simulink model "manchestermodelcommblks"  (Simulink 5.1)
settings: Solver=FixedStepDiscrete  SolverMode=SingleTasking  StartTime=0.0  StopTime=50000  RelTol=1e-3
undefined symbols (not defined in the file or in its folder): sigbuilder_block
libraries: fixpt_lib_4 x6, dspsigops x5, commsink2 x2, dspswit3 x1, dspsrcs4 x1, simulink x1, modelsimlib x1
settings Model: Creator=adowd  LastModifiedBy=nsen  ExtModeAutoUpdateStatusClock=off  SaveTime=off  SaveOutput=off  BooleanDataType=on  ProdHWDeviceType=Microprocessor  RTWOptions="-aEnforceIntegerDowncast=1 -aExtMode=0 -aExtModeTesting=0 -aFoldNonRolledExpr=1 -aForceParamTrailComments=0 -aGenerateComments=1 -aGenerateReport=0 -aIgnoreCustomStorageClasses=1 -aIncDataTypeInIds=0 -aIncHierarchyInIds=0 -aInlineInvariantSignals=0 -aInlinedPrmAccess=\"Literals\" -aLocalBlockOutputs=1 -aLogVarNameModifier=\"rt_\" -aMaxRTWIdLen=31 -aPrefixModelToSubsysFcnNames=1 -aRTWVerbose=1 -aRollThreshold=5 -aShowEliminatedStatements=0"

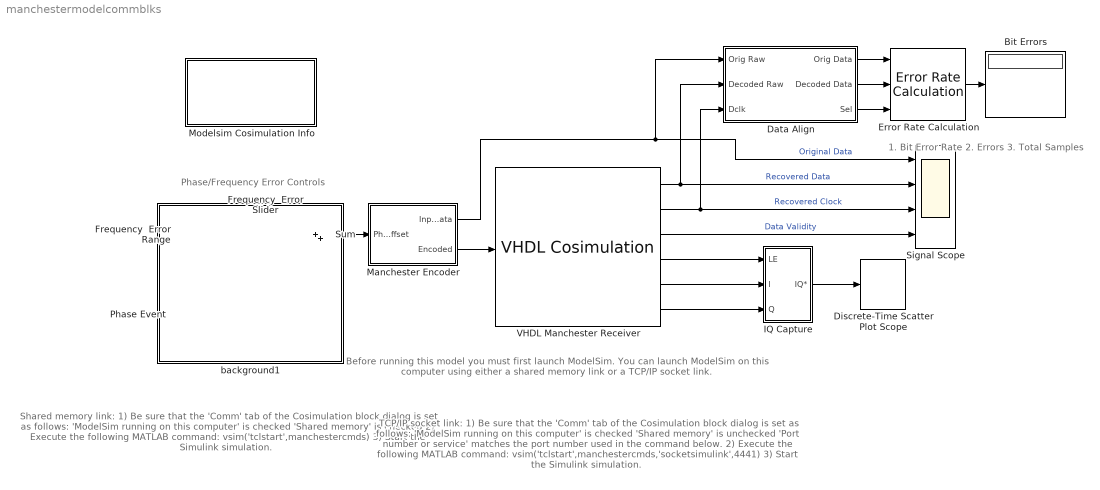
== system manchestermodelcommblks ==
  note: Phase/Frequency Error Controls
  note: 1. Bit Error Rate
      | 2. Errors
      | 3. Total Samples
  note: Before running this model you must first launch ModelSim.
      | You can launch ModelSim on this computer using either a
      | shared memory link or a TCP/IP socket link.
  note: Shared memory link:
      |     1) Be sure that the 'Comm' tab of the Cosimulation block
      |          dialog is set as follows:
      |             'ModelSim running on this computer' is checked
      |             'Shared memory' is checked
      |     2) Execute the following MATLAB command:
      |             vsim('tclstart',manchestercmds)
      |     3) Start the Simulink simulation.
  note: TCP/IP socket link:
      |     1) Be sure that the 'Comm' tab of the Cosimulation block
      |          dialog is set as follows:
      |             'ModelSim running on this computer' is checked
      |             'Shared memory' is unchecked
      |             'Port number or service' matches the port number used
      |                    in the command below.
      |     2) Execute the following MATLAB command:
      |             vsim('tclstart',manchestercmds,'socketsimulink',4441)
      |     3) Start the Simulink simulation.
  Bit Errors : Display
  Data Align : Subsystem
  Discrete-Time Scatter Plot Scope : commsink2/Discrete-Time Scatter Plot Scope  Tag=ScatterPlot  showPlotting=on  sampPerSymb=1  offsetEye=0  numTraces=256  numNewFrames=32  showRendering=on  LineMarkers=d  LineColors=b  fading=on  render=off  AxisGrid=on  showAxes=off  xMin=-0.82  xMax=16.82  yMin=-0.800000000000001  yMax=16.84  inphaseLabel=In-phase Amplitude  quadratureLabel=Quadrature Amplitude  showFigure=off  openScopeAtSimStart=on  FrameNumber=off  FigPos=[360 532 402 402]  figTitle=IQ Measurements  numLinesMax=8  block_type_=scatter
  Error Rate Calculation : commsink2/Error Rate Calculation  N=0  st_delay=0  cp_mode=Select samples from port  subframe=[]  PMode=Port  WsName=ErrorVec  RsMode2=off  stop=off  numErr=100  maxBits=1e6
  Frequency  Error Range : dspsrcs4/DSP Constant  Value=1/128  SampleMode=Discrete  discreteOutput=Sample-based  continuousOutput=Sample-based  sampTime=10  framePeriod=2  dataType=Inherit from 'Constant value'  wordLen=16  udDataType=sfix(16)  fracBitsMode=Best precision  numFracBits=15  InterpretAs1D=-inf  Ts=-inf  FramebasedOutput=-inf
  Frequency  Error Slider : simulink/Math Operations/Slider Gain  low=-1  gain=0  high=1
  IQ Capture : Subsystem
  Manchester Encoder : Subsystem
  Modelsim Cosimulation Info : Subsystem
      mask Type: VHDL Manchester Receiver Demo Info
      mask Display: disp('VHDL Manchester\nReceiver Simulation\nInformation')
  Phase Event : Subsystem  Tag=STV Subsys  StartFcn=sigbuilder_block('start');  StopFcn=sigbuilder_block('stop');  ClipboardFcn=sigbuilder_block('clipboard');  mask(Sigbuilder block){}
      mask help: Sigbuilder GUI
      mask init:
      | if ~strcmp(get_param(bdroot(gcb),'SimulationStatus'),'stopped') tuvar = sigbuilder_block('maskInit'); end
      settings: CopyFcn=sigbuilder_block('copy');  DeleteFcn=sigbuilder_block('delete');  ModelCloseFcn=sigbuilder_block('modelClose');  PreSaveFcn=sigbuilder_block('preSave');  NameChangeFcn=sigbuilder_block('namechange');  OpenFcn=sigbuilder_block('open',[172.5 90 733.5 575.25 ]);  CloseFcn=sigbuilder_block('close');
      mask Display: plot(0,0,100,100,[10,10,40,40,10],[80,20,20,80,80],[40,10],[50,50], [40,27,10],[65,72,56],[40,25,25,10],[28,28,43,43]);
  Signal Scope : Scope  NumInputPorts=4
      settings: TimeRange=3000  YMin=-1~-1~-1~0.95  YMax=2~2~2~1.05
  Sum : Sum  Inputs=|++  SaturateOnIntegerOverflow=on
  VHDL Manchester Receiver : modelsimlib/VHDL Cosimulation  idxCellArray={'/manchester/samp', 'in', '/manchester/data', 'out', '/manchester/dclk', 'out', '/manchester/dvalid', 'out', '/manchester/sync_i', 'out', '/manchester/isum_i', 'out', '/manchester/qsum_i', 'out', '/manchester/clk', 'rclk'}  Tso=-1  tclBefore=force /manchester/enable 1 0; force sim:/manchester/reset 1 0, 0 1000 ns  tclAfter="echo \"done\""  hostName='modelsim_comp'  portNumber=4441  modelSimRunning=on  sharedMemory=on
  background1 : Subsystem
      mask Display: disp('')
  wires:
  Manchester Encoder/2(Encoded) -> VHDL Manchester Receiver/1
  VHDL Manchester Receiver/3 -> Signal Scope/4  "Data Validity"
  Sum/1 -> Manchester Encoder/1(Phase Offset)
  Phase Event/1(Phase) -> Sum/2
  VHDL Manchester Receiver/2 -> Signal Scope/3, Data Align/3(Dclk)  "Recovered Clock"
  Error Rate Calculation/1 -> Bit Errors/1
  Data Align/1(Orig Data) -> Error Rate Calculation/1
  Data Align/2(Decoded Data) -> Error Rate Calculation/2
  Manchester Encoder/1(Input Data) -> Data Align/1(Orig Raw), Signal Scope/1  "Original Data"
  IQ Capture/1(IQ*) -> Discrete-Time Scatter Plot Scope/1
  Frequency  Error Range/1 -> Frequency  Error Slider/1
  Frequency  Error Slider/1 -> Sum/1
  VHDL Manchester Receiver/1 -> Signal Scope/2, Data Align/2(Decoded Raw)  "Recovered Data"
  Data Align/3(Sel) -> Error Rate Calculation/3
  VHDL Manchester Receiver/4 -> IQ Capture/1(LE)
  VHDL Manchester Receiver/6 -> IQ Capture/3(Q)
  VHDL Manchester Receiver/5 -> IQ Capture/2(I)

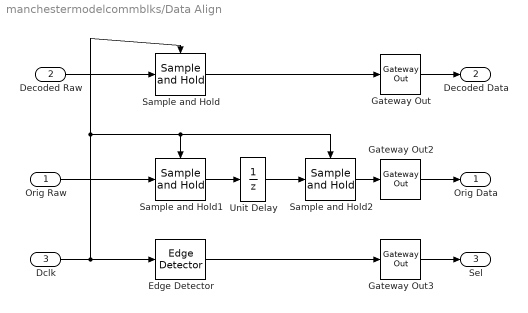
== system manchestermodelcommblks/Data Align ==
  Orig Raw : Inport
  Decoded Raw : Inport  Port=2
  Dclk : Inport  Port=3
  Edge Detector : dspswit3/Edge Detector
  Gateway Out : fixpt_lib_4/Data Type/Gateway Out  OutRealWorld=Real World Value  OutBuiltInType=double  RndMeth=Nearest  DoSatur=off
  Gateway Out2 : fixpt_lib_4/Data Type/Gateway Out  OutRealWorld=Real World Value  OutBuiltInType=double  RndMeth=Nearest  DoSatur=off
  Gateway Out3 : fixpt_lib_4/Data Type/Gateway Out  OutRealWorld=Real World Value  OutBuiltInType=double  RndMeth=Nearest  DoSatur=off
  Sample and Hold : dspsigops/Sample and Hold  trig=Rising edge  initCond=0
  Sample and Hold1 : dspsigops/Sample and Hold  trig=Rising edge  initCond=0
  Sample and Hold2 : dspsigops/Sample and Hold  trig=Rising edge  initCond=0
  Unit Delay : UnitDelay  X0=0.0  SampleTime=-1
  Orig Data : Outport
  Decoded Data : Outport  Port=2
  Sel : Outport  Port=3
  wires:
  Sample and Hold1/1 -> Unit Delay/1
  Decoded Raw/1 -> Sample and Hold/1
  Dclk/1 -> Sample and Hold/Trigger, Sample and Hold1/Trigger, Sample and Hold2/Trigger, Edge Detector/1
  Orig Raw/1 -> Sample and Hold1/1
  Sample and Hold/1 -> Gateway Out/1
  Unit Delay/1 -> Sample and Hold2/1
  Sample and Hold2/1 -> Gateway Out2/1
  Edge Detector/1 -> Gateway Out3/1
  Gateway Out3/1 -> Sel/1
  Gateway Out/1 -> Decoded Data/1
  Gateway Out2/1 -> Orig Data/1

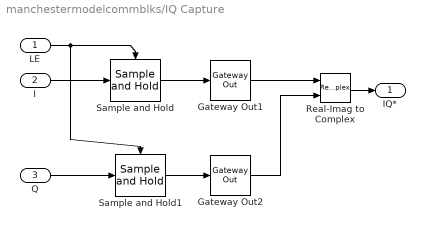
== system manchestermodelcommblks/IQ Capture ==
  LE : Inport
  I : Inport  Port=2
  Q : Inport  Port=3
  Gateway Out1 : fixpt_lib_4/Data Type/Gateway Out  OutRealWorld=Real World Value  OutBuiltInType=double  RndMeth=Nearest  DoSatur=off
  Gateway Out2 : fixpt_lib_4/Data Type/Gateway Out  OutRealWorld=Real World Value  OutBuiltInType=double  RndMeth=Nearest  DoSatur=off
  Real-Imag to Complex : RealImagToComplex
  Sample and Hold : dspsigops/Sample and Hold  trig=Rising edge  initCond=0
  Sample and Hold1 : dspsigops/Sample and Hold  trig=Rising edge  initCond=0
  IQ* : Outport
  wires:
  LE/1 -> Sample and Hold/Trigger, Sample and Hold1/Trigger
  Sample and Hold/1 -> Gateway Out1/1
  Sample and Hold1/1 -> Gateway Out2/1
  Gateway Out1/1 -> Real-Imag to Complex/1
  Gateway Out2/1 -> Real-Imag to Complex/2
  I/1 -> Sample and Hold/1
  Real-Imag to Complex/1 -> IQ*/1
  Q/1 -> Sample and Hold1/1

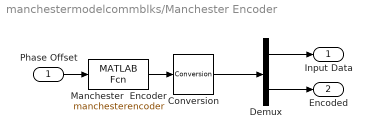
== system manchestermodelcommblks/Manchester Encoder ==
  Phase Offset : Inport
  Conversion : fixpt_lib_4/Data Type/Conversion  ConvertRealWorld=Real World Value  OutputDataTypeScalingMode=Specify via dialog  OutDataType=ufix(1)  OutScaling=1  DoSatur=off
  Demux : Demux  Outputs=2
  Manchester  Encoder : MATLABFcn  MATLABFcn=manchesterencoder
  Input Data : Outport
  Encoded : Outport  Port=2
  wires:
  Manchester  Encoder/1 -> Conversion/1
  Conversion/1 -> Demux/1
  Demux/1 -> Input Data/1
  Phase Offset/1 -> Manchester  Encoder/1
  Demux/2 -> Encoded/1

== system manchestermodelcommblks/Modelsim Cosimulation Info ==
  note: Manchester Recevier
      |
      |
      | Manchester encoding is a simple modulation scheme that converts baseband digital
      | data to an encoded waveform with no DC component.  The most widely known
      | application of this technique is Ethernet.
      |
      | This model simulates a digital receiver of Manchester encoded data.  The receiver is
      | implemented in VHDL.  The  receiver uses a simple DLL (delay lock loop) clock recovery
      | mechanism, which requires multiple cycles to lock with the incoming data stream.  The
      | performance of the receiver is explored by applying phase and frequency errors to a randomly
      | generated stream of bits that is encoded using a simple MATLAB function: manchesterencoder().
      |
      |  The VHDL code runs in ModelSim as a ModelSim VHDL Cosimulation block
      | labeled VHDL Manchester Receiver.

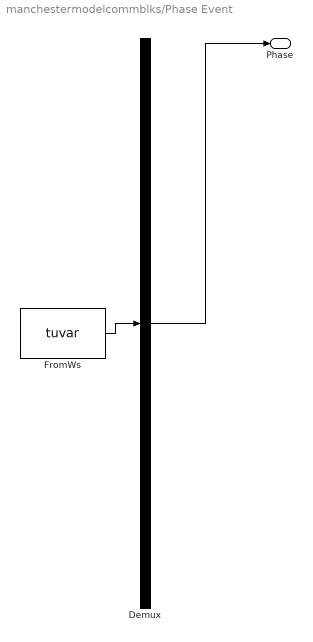
== system manchestermodelcommblks/Phase Event ==
  Demux : Demux  Tag=STV Demux  Outputs=1
  FromWs : FromWorkspace  Tag=STV FromWs  VariableName=tuvar  SampleTime=10  OutputAfterFinalValue=Holding final value  SigBuilderData=DataTag0
      SigBuilderData=|
      | channels.label = 'Phase'
      | channels.allXData = {[0 10055 10055 10410 10410 30000]}
      | channels.allYData = {[0 0 0.0764 0.0764 0 0]}
      | common.afterFinalStr = 'Hold final value'
      | common.sampleTime = 10
      | dataSet.timeRange = [0 30000]
      | dataSet.name = 'Group 1'
  Phase : Outport  Tag=STV Outport
  wires:
  Demux/1 -> Phase/1
  FromWs/1 -> Demux/1

== system manchestermodelcommblks/background1 ==
